simulink model "cps_log_video_v2"  (R2012b)
settings: Solver=FixedStepDiscrete  StartTime=0.0  StopTime=8.5  RelTol=20e-5
model workspace (MAT data in the model file):
  ini_block_hpos = -0.4
  ini_block_vpos = 0.11
  ini_nozzle_vpos = 0.3
settings Model: Creator=pmosterm  LastModifiedBy=pmosterm
settings SolverCC: ZcThreshold=2e-5  MaxConsecutiveZCs=20  EnableConcurrentExecution=on  ConcurrentTasks=on  ZeroCrossAlgorithm=Adaptive  SolverResetMethod=Robust
settings DataIOCC: SignalLoggingSaveFormat=ModelDataLogs
settings OptimizationCC: InlineParams=on
settings DebuggingCC: AlgebraicLoopMsg=error  UnderspecifiedInitializationDetection=Simplified  FcnCallInpInsideContextMsg=EnableAllAsWarning  ModelReferenceExtraNoncontSigs=warning
settings ModelReferenceCC: ModelReferenceNumInstancesAllowed=Single
settings GRTTargetCC: CombineOutputUpdateFcns=off  GRTInterface=on
settings ConfigurationSet: Description=SimMechanics 2G

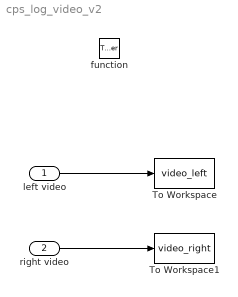
== system cps_log_video_v2 ==
  left video : Inport  OutDataTypeStr=uint8  PortDimensions=[400 240 3]
  right video : Inport  Port=2  OutDataTypeStr=uint8  PortDimensions=[400 240 3]
  function : TriggerPort  TriggerType=function-call
  To Workspace : ToWorkspace  VariableName=video_left  SampleTime=-1
  To Workspace1 : ToWorkspace  VariableName=video_right  SampleTime=-1
  wires:
  left video/1 -> To Workspace/1
  right video/1 -> To Workspace1/1
